simulink model "Microgrid_transition_model_092221"  (R2020a)
settings: Solver=VariableStepAuto  StartTime=0.0  StopTime=16  MaxStep=1e-4  RelTol=1e-3
PreLoadFcn:
  | %run('FC_microgrid_param.m')
  | %load('gen_grid_init.mat')
InitFcn:
  | %load myisoModel_init;
  | run('FC_microgrid_param.m')
  | tic
  | run('CARTinitFcn.m')
  | %caseNo = 2;
  | 
  | %if (caseNo == 1)
  | %set_param(['Isolated_grid_paper_model_022521/SignalGen'], 'ActiveScenario', 'PStep222kW');
  | %else
  | %set_param(['Isolated_grid_paper_model_022521/SignalGen'], 'ActiveScenario', 'QStep222kVAr');
  | 
  | %end;
StopFcn:
  | toc
undefined symbols (not defined in the file): breakpoints1, breakpoints2, cp_table_data, ctrl, D1, Delta, DiscIntNeverNeededParam, DT, FC_BESS, find_system, gcbh, libFC_BESS, LowerLimit, magnitude, oversize, pq_ts, sps_rtmsupport, timer, ts, Ts, Ts_APC, Ts_Control, Ts_Power, UpperLimit
libraries: powerlib x120, powerlib_meascontrol x85, simulink x63, powerlib_extras x40, simulink_extras x12, eePowerMeasurement x9, sps_avr x7, pi_ctrl x4, spsDieselMotorModel x3, SignalEditorBlockLib x2, libLgBattery x1, libFC_PV x1
(part 6 of 11)

== system Microgrid_transition_model_092221/Defferable Load (0-446.25 kW)/Switches/Switches ABC5 ==
  P_ABC : Inport
  Demux : Demux  Outputs=3
      settings: DisplayOption=none
  Switch A : powerlib/Power Electronics/Ideal Switch  Ron=Ron_switch  Lon=0  IC=Status(6)  Rs=Rs_snubber  Cs=Cs_snubber  Measurements=off
      settings: AttributesFormatString=\n  SourceProductBaseCode=MT,PS
  Switch B : powerlib/Power Electronics/Ideal Switch  Ron=Ron_switch  Lon=0  IC=Status(6)  Rs=Rs_snubber  Cs=Cs_snubber  Measurements=off
      settings: AttributesFormatString=\n  SourceProductBaseCode=MT,PS
  Switch C : powerlib/Power Electronics/Ideal Switch  Ron=Ron_switch  Lon=0  IC=Status(6)  Rs=Rs_snubber  Cs=Cs_snubber  Measurements=off
      settings: AttributesFormatString=\n  SourceProductBaseCode=MT,PS
  A : PMIOPort  Side=Left
  B : PMIOPort  Port=2  Side=Left
  C : PMIOPort  Port=3  Side=Left
  "A " : PMIOPort  Port=4  Side=Right
  "B " : PMIOPort  Port=5  Side=Right
  "C " : PMIOPort  Port=6  Side=Right
  wires:
  Demux/1 -> Switch A/1
  Demux/2 -> Switch B/1
  Demux/3 -> Switch C/1
  P_ABC/1 -> Demux/1
  connections:
  C/RConn1 -- Switch C/LConn1
  B/RConn1 -- Switch B/LConn1
  A/RConn1 -- Switch A/LConn1
  Switch A/RConn1 -- "A "/RConn1
  Switch B/RConn1 -- "B "/RConn1
  Switch C/RConn1 -- "C "/RConn1

== system Microgrid_transition_model_092221/Defferable Load (0-446.25 kW)/Switches/Switches ABC6 ==
  P_ABC : Inport
  Demux : Demux  Outputs=3
      settings: DisplayOption=none
  Switch A : powerlib/Power Electronics/Ideal Switch  Ron=Ron_switch  Lon=0  IC=Status(7)  Rs=Rs_snubber  Cs=Cs_snubber  Measurements=off
      settings: AttributesFormatString=\n  SourceProductBaseCode=MT,PS
  Switch B : powerlib/Power Electronics/Ideal Switch  Ron=Ron_switch  Lon=0  IC=Status(7)  Rs=Rs_snubber  Cs=Cs_snubber  Measurements=off
      settings: AttributesFormatString=\n  SourceProductBaseCode=MT,PS
  Switch C : powerlib/Power Electronics/Ideal Switch  Ron=Ron_switch  Lon=0  IC=Status(7)  Rs=Rs_snubber  Cs=Cs_snubber  Measurements=off
      settings: AttributesFormatString=\n  SourceProductBaseCode=MT,PS
  A : PMIOPort  Side=Left
  B : PMIOPort  Port=2  Side=Left
  C : PMIOPort  Port=3  Side=Left
  "A " : PMIOPort  Port=4  Side=Right
  "B " : PMIOPort  Port=5  Side=Right
  "C " : PMIOPort  Port=6  Side=Right
  wires:
  P_ABC/1 -> Demux/1
  Demux/3 -> Switch C/1
  Demux/2 -> Switch B/1
  Demux/1 -> Switch A/1
  connections:
  Switch C/RConn1 -- "C "/RConn1
  Switch B/RConn1 -- "B "/RConn1
  Switch A/RConn1 -- "A "/RConn1
  A/RConn1 -- Switch A/LConn1
  B/RConn1 -- Switch B/LConn1
  C/RConn1 -- Switch C/LConn1

== system Microgrid_transition_model_092221/Defferable Load (0-446.25 kW)/Switches/Switches ABC7 ==
  P_ABC : Inport
  Demux : Demux  Outputs=3
      settings: DisplayOption=none
  Switch A : powerlib/Power Electronics/Ideal Switch  Ron=Ron_switch  Lon=0  IC=Status(8)  Rs=Rs_snubber  Cs=Cs_snubber  Measurements=off
      settings: AttributesFormatString=\n  SourceProductBaseCode=MT,PS
  Switch B : powerlib/Power Electronics/Ideal Switch  Ron=Ron_switch  Lon=0  IC=Status(8)  Rs=Rs_snubber  Cs=Cs_snubber  Measurements=off
      settings: AttributesFormatString=\n  SourceProductBaseCode=MT,PS
  Switch C : powerlib/Power Electronics/Ideal Switch  Ron=Ron_switch  Lon=0  IC=Status(8)  Rs=Rs_snubber  Cs=Cs_snubber  Measurements=off
      settings: AttributesFormatString=\n  SourceProductBaseCode=MT,PS
  A : PMIOPort  Side=Left
  B : PMIOPort  Port=2  Side=Left
  C : PMIOPort  Port=3  Side=Left
  "A " : PMIOPort  Port=4  Side=Right
  "B " : PMIOPort  Port=5  Side=Right
  "C " : PMIOPort  Port=6  Side=Right
  wires:
  Demux/1 -> Switch A/1
  Demux/2 -> Switch B/1
  Demux/3 -> Switch C/1
  P_ABC/1 -> Demux/1
  connections:
  C/RConn1 -- Switch C/LConn1
  B/RConn1 -- Switch B/LConn1
  A/RConn1 -- Switch A/LConn1
  Switch A/RConn1 -- "A "/RConn1
  Switch B/RConn1 -- "B "/RConn1
  Switch C/RConn1 -- "C "/RConn1

== system Microgrid_transition_model_092221/FC_BESS/SMAInverter/85_SMAControl ==
  Uabc : Inport
  Uabc_inv : Inport  Port=2
  Iabc : Inport  Port=3
  CB_status : Inport  Port=4
  Control : Inport  Port=5
  Bus Creator1 : BusCreator  Inputs=2
  Bus Creator5 : BusCreator  Inputs=1
  Bus Selector : BusSelector  OutputSignals=p_ref,q_ref,f_ref,v_ref,GF_mode
  InvControl : Subsystem  mask{Ts=Ts_Control, Unpp=400, Pn=1e6}
      mask prompts: Ts "Control sample time [s]"; Unpp "Nominal AC voltage [Vpp]"; Pn "Nominal Power [W]"
      mask init:
      | Unom = Unpp / sqrt(3);
      | Inom = Pn/3/Unom;
  Rate Transition{,1..2,4..7,9..10} (9 alike) : RateTransition  Integrity=off  OutPortSampleTime=Ts_Control
  Rate Transition3 : RateTransition  OutPortSampleTime=Ts
  Rate Transition8 : RateTransition  OutPortSampleTime=Ts
  Scope : Scope
  Step : Step  Before=1  After=0  SampleTime=Ts
  Step1 : Step  Time=98  SampleTime=Ts
  Sum : Sum  Inputs=|++
  CtrlOut : Outport
  wires:
  Rate Transition4/1 -> InvControl/5(pref)
  Iabc/1 -> Rate Transition1/1
  Rate Transition2/1 -> InvControl/4(cb_stat)
  Rate Transition1/1 -> InvControl/3(Iabc)
  Rate Transition/1 -> InvControl/1(Uabc)
  Rate Transition8/1 -> Bus Creator5/1  "Close"
  Step/1 -> Sum/1
  InvControl/1(Uabc_ref) -> Rate Transition3/1
  Rate Transition3/1 -> Bus Creator1/1  "Uabc"
  Uabc/1 -> Rate Transition/1
  CB_status/1 -> Rate Transition2/1
  Bus Creator5/1 -> Bus Creator1/2  "ToCB"
  Bus Creator1/1 -> CtrlOut/1
  Bus Selector/1 -> Rate Transition4/1  "<p_ref>"
  Bus Selector/2 -> Rate Transition5/1  "<q_ref>"
  Bus Selector/3 -> Rate Transition6/1  "<f_ref>"
  Bus Selector/4 -> Rate Transition7/1  "<v_ref>"
  Bus Selector/5 -> Rate Transition9/1  "<GF_mode>"
  Rate Transition9/1 -> InvControl/9(GF_mode_en)
  Rate Transition7/1 -> InvControl/8(vref)
  Rate Transition5/1 -> InvControl/6(qref)
  Rate Transition6/1 -> InvControl/7(fref)
  Control/1 -> Bus Selector/1
  Uabc_inv/1 -> Rate Transition10/1
  Rate Transition10/1 -> InvControl/2(Uabc_inv)
  Step1/1 -> Sum/2
  Sum/1 -> Scope/1, Rate Transition8/1

== system Microgrid_transition_model_092221/FC_BESS/SMAInverter/BESS Inverter ==
  ctrl : Inport
  Controlled Voltage Source : powerlib/Electrical Sources/Controlled Voltage Source  Initialize=on  Source_Type=AC  Amplitude=0  Phase=0  Frequency=0  Measurements=None
  Controlled Voltage Source1 : powerlib/Electrical Sources/Controlled Voltage Source  Initialize=on  Source_Type=AC  Amplitude=0  Phase=0  Frequency=0  Measurements=None
  Controlled Voltage Source2 : powerlib/Electrical Sources/Controlled Voltage Source  Initialize=on  Source_Type=AC  Amplitude=0  Phase=0  Frequency=0  Measurements=None
  Demux : Demux  Outputs=3
  A : PMIOPort  Side=Right
  N : PMIOPort  Port=2  Side=Left
  B : PMIOPort  Port=3  Side=Right
  C : PMIOPort  Port=4  Side=Right
  wires:
  ctrl/1 -> Demux/1
  Demux/3 -> Controlled Voltage Source2/1
  Demux/2 -> Controlled Voltage Source1/1
  Demux/1 -> Controlled Voltage Source/1
  connections:
  Controlled Voltage Source2/RConn1 -- C/RConn1
  Controlled Voltage Source1/RConn1 -- B/RConn1
  N/RConn1 -- Controlled Voltage Source1/LConn1 -- Controlled Voltage Source/LConn1 -- Controlled Voltage Source2/LConn1
  A/RConn1 -- Controlled Voltage Source/RConn1

== system Microgrid_transition_model_092221/FC_BESS/SMAInverter/Subsystem ==
  GRI1 : powerlib/Measurements/Three-Phase V-I Measurement  VoltageMeasurement=phase-to-ground  SetLabelV=off  LabelV=Ugri  Vpu=off  VpuLL=off  CurrentMeasurement=yes  SetLabelI=off  LabelI=Igri  Ipu=off  Pbase=100e6  Vbase=500e3  OutputType=Complex  PhasorSimulation=off  PSBequivalent=0
  A : PMIOPort  Side=Left
  B : PMIOPort  Port=2  Side=Left
  a : PMIOPort  Port=3  Side=Right
  b : PMIOPort  Port=4  Side=Right
  C : PMIOPort  Port=5  Side=Left
  c : PMIOPort  Port=6  Side=Right
  tag scope: Igri=scoped, Ugri=scoped
  wires:
  GRI1/2 -> [Igri]
  GRI1/1 -> [Ugri]
  connections:
  GRI1/RConn1 -- a/RConn1
  GRI1/LConn1 -- A/RConn1
  GRI1/RConn2 -- b/RConn1
  GRI1/RConn3 -- c/RConn1
  GRI1/LConn2 -- B/RConn1
  GRI1/LConn3 -- C/RConn1

== system Microgrid_transition_model_092221/FC_BESS/SMAInverter/Subsystem1 ==
  SmaINV : powerlib/Measurements/Three-Phase V-I Measurement  VoltageMeasurement=phase-to-ground  SetLabelV=off  LabelV=circuit_Usmainv  Vpu=off  VpuLL=off  CurrentMeasurement=yes  SetLabelI=off  LabelI=circuit_Ismainv  Ipu=off  Pbase=100e6  Vbase=500e3  OutputType=Complex  PhasorSimulation=off  PSBequivalent=0
  A : PMIOPort  Side=Left
  a : PMIOPort  Port=2  Side=Right
  B : PMIOPort  Port=3  Side=Left
  b : PMIOPort  Port=4  Side=Right
  C : PMIOPort  Port=5  Side=Left
  c : PMIOPort  Port=6  Side=Right
  tag scope: Iinv=scoped, Uinv=scoped
  wires:
  SmaINV/1 -> [Uinv]
  SmaINV/2 -> [Iinv]
  connections:
  SmaINV/RConn1 -- a/RConn1
  C/RConn1 -- SmaINV/LConn3
  SmaINV/LConn2 -- B/RConn1
  SmaINV/RConn2 -- b/RConn1
  SmaINV/RConn3 -- c/RConn1
  A/RConn1 -- SmaINV/LConn1

== system Microgrid_transition_model_092221/Grid Feeder Protective Relay/CS Modified PLL/Controller ==
  note: Pierre Giroux, Gilbert Sybille
      | Power System Simulation Laboratory
      | IREQ, Hydro-Quebc
  note: Discrete PID Controller
  Error : Inport
  Discrete Derivative : simulink/Discrete/Discrete Derivative  gainval=1.0  ICPrevScaledInput=0.0  OutMin=[]  OutMax=[]  OutDataType=sfix(16)  OutScaling=2^-10  DoSatur=off
  Discrete-Time Integrator : DiscreteIntegrator  InitialCondition=Init  SampleTime=Ts  LimitOutput=on  UpperSaturationLimit=UpperLimit  LowerSaturationLimit=LowerLimit  ICPrevOutput=DiscIntNeverNeededParam  ICPrevScaledInput=DiscIntNeverNeededParam
  Kp4 : Gain  Gain=Kp  SaturateOnIntegerOverflow=on  OutDataTypeStr=Inherit: Same as input  ParamDataTypeStr=Inherit: Same as input
  Kp5 : Gain  Gain=Ki  SaturateOnIntegerOverflow=on  OutDataTypeStr=Inherit: Same as input  ParamDataTypeStr=Inherit: Same as input
  Kp6 : Gain  Gain=Kd  SaturateOnIntegerOverflow=on  OutDataTypeStr=Inherit: Same as input  ParamDataTypeStr=Inherit: Same as input
  Saturation2 : Saturate  UpperLimit=UpperLimit  LowerLimit=LowerLimit
  Sum6 : Sum  Inputs=+++  InputSameDT=on  SaturateOnIntegerOverflow=on  OutDataTypeStr=Inherit: Same as first input
  Zero-Order Hold : ZeroOrderHold  SampleTime=Ts
  Out : Outport  InitialOutput=0
  wires:
  Error/1 -> Kp4/1, Kp5/1, Kp6/1
  Sum6/1 -> Saturation2/1
  Kp5/1 -> Discrete-Time Integrator/1
  Kp6/1 -> Zero-Order Hold/1
  Kp4/1 -> Sum6/1
  Discrete-Time Integrator/1 -> Sum6/2
  Discrete Derivative/1 -> Sum6/3
  Saturation2/1 -> Out/1
  Zero-Order Hold/1 -> Discrete Derivative/1

== system Microgrid_transition_model_092221/Grid Feeder Protective Relay/CS Modified PLL/VCO ==
  w : Inport
  Compare To Constant : simulink/Logic and Bit Operations/Compare To Constant  relop=>=  const=pi  OutDataTypeStr=uint8
  Gain : Gain  Gain=2*pi  OutDataTypeStr=double
  Gain2 : Gain  Gain=Ts  SaturateOnIntegerOverflow=on  OutDataTypeStr=Inherit: Same as input  ParamDataTypeStr=Inherit: Same as input
  Sum : Sum  Inputs=-++
  Unit Delay1 : UnitDelay  SampleTime=-1  HasFrameUpgradeWarning=on
  theta : Outport
  wires:
  w/1 -> Gain2/1
  Gain/1 -> Sum/1
  Compare To Constant/1 -> Gain/1
  Unit Delay1/1 -> Compare To Constant/1, Sum/3, theta/1  "wt"
  Gain2/1 -> Sum/2
  Sum/1 -> Unit Delay1/1

== system Microgrid_transition_model_092221/Grid Feeder Protective Relay/CS Modified PLL1/Controller ==
  note: Pierre Giroux, Gilbert Sybille
      | Power System Simulation Laboratory
      | IREQ, Hydro-Quebc
  note: Discrete PID Controller
  Error : Inport
  Discrete Derivative : simulink/Discrete/Discrete Derivative  gainval=1.0  ICPrevScaledInput=0.0  OutMin=[]  OutMax=[]  OutDataType=sfix(16)  OutScaling=2^-10  DoSatur=off
  Discrete-Time Integrator : DiscreteIntegrator  InitialCondition=Init  SampleTime=Ts  LimitOutput=on  UpperSaturationLimit=UpperLimit  LowerSaturationLimit=LowerLimit  ICPrevOutput=DiscIntNeverNeededParam  ICPrevScaledInput=DiscIntNeverNeededParam
  Kp4 : Gain  Gain=Kp  SaturateOnIntegerOverflow=on  OutDataTypeStr=Inherit: Same as input  ParamDataTypeStr=Inherit: Same as input
  Kp5 : Gain  Gain=Ki  SaturateOnIntegerOverflow=on  OutDataTypeStr=Inherit: Same as input  ParamDataTypeStr=Inherit: Same as input
  Kp6 : Gain  Gain=Kd  SaturateOnIntegerOverflow=on  OutDataTypeStr=Inherit: Same as input  ParamDataTypeStr=Inherit: Same as input
  Saturation2 : Saturate  UpperLimit=UpperLimit  LowerLimit=LowerLimit
  Sum6 : Sum  Inputs=+++  InputSameDT=on  SaturateOnIntegerOverflow=on  OutDataTypeStr=Inherit: Same as first input
  Zero-Order Hold : ZeroOrderHold  SampleTime=Ts
  Out : Outport  InitialOutput=0
  wires:
  Error/1 -> Kp4/1, Kp5/1, Kp6/1
  Sum6/1 -> Saturation2/1
  Kp5/1 -> Discrete-Time Integrator/1
  Kp6/1 -> Zero-Order Hold/1
  Kp4/1 -> Sum6/1
  Discrete-Time Integrator/1 -> Sum6/2
  Discrete Derivative/1 -> Sum6/3
  Saturation2/1 -> Out/1
  Zero-Order Hold/1 -> Discrete Derivative/1

== system Microgrid_transition_model_092221/Grid Feeder Protective Relay/CS Modified PLL1/VCO ==
  w : Inport
  Compare To Constant : simulink/Logic and Bit Operations/Compare To Constant  relop=>=  const=pi  OutDataTypeStr=uint8
  Gain : Gain  Gain=2*pi  OutDataTypeStr=double
  Gain2 : Gain  Gain=Ts  SaturateOnIntegerOverflow=on  OutDataTypeStr=Inherit: Same as input  ParamDataTypeStr=Inherit: Same as input
  Sum : Sum  Inputs=-++
  Unit Delay1 : UnitDelay  SampleTime=-1  HasFrameUpgradeWarning=on
  theta : Outport
  wires:
  w/1 -> Gain2/1
  Gain/1 -> Sum/1
  Compare To Constant/1 -> Gain/1
  Unit Delay1/1 -> Compare To Constant/1, Sum/3, theta/1  "wt"
  Gain2/1 -> Sum/2
  Sum/1 -> Unit Delay1/1

== system Microgrid_transition_model_092221/Grid Feeder Protective Relay/R25 - Sync Check v0.1/Freq_Comparator ==
  note: This block compares the frequency at the circuit breaker terminals
      | * if the difference is less than threshold dF_threshold, then outputs 1
  f_grid : Inport
  f_gen : Inport  Port=2
  dF_threshold : Inport  Port=3
  Fcn2 : Fcn  Expr=abs(u(2)-u(1)) <= u(3)
  Mux1 : Mux  Inputs=3
  Sum : Sum  Inputs=+-
  Locked : Outport
  dF : Outport  Port=2
  wires:
  Sum/1 -> dF/1
  f_grid/1 -> Mux1/1, Sum/2
  f_gen/1 -> Mux1/2, Sum/1
  dF_threshold/1 -> Mux1/3
  Fcn2/1 -> Locked/1
  Mux1/1 -> Fcn2/1

== system Microgrid_transition_model_092221/Grid Feeder Protective Relay/R25 - Sync Check v0.1/Phase_Comparator ==
  note: This block compares the angle (phase A only) at the circuit breaker terminals
      | * if the difference is less than threshold angle_threshold, then outputs 1
  wt_grid : Inport
  wt_gen : Inport  Port=2
  angle_threshold : Inport  Port=3
  Abs : Abs
  Fcn1 : Fcn  Expr=u(1) <= u(2)  SampleTime=Ts
  Mux1 : Mux  Inputs=2
  Radians to Degrees : simulink_extras/Transformations/Radians to Degrees
  Scope : Scope
  Sum1 : Sum  Inputs=|-+
  WrapPi : Subsystem
  Locked : Outport
  dWt : Outport  Port=2
  wires:
  WrapPi/1(Out1) -> Abs/1, dWt/1
  Sum1/1 -> WrapPi/1(In1)
  wt_grid/1 -> Sum1/1
  wt_gen/1 -> Sum1/2
  Radians to Degrees/1 -> Scope/1, Mux1/1  "R2D"
  Mux1/1 -> Fcn1/1
  angle_threshold/1 -> Mux1/2
  Fcn1/1 -> Locked/1  "bool"
  Abs/1 -> Radians to Degrees/1  "diff"

== system Microgrid_transition_model_092221/Grid Feeder Protective Relay/R25 - Sync Check v0.1/Voltage_Comparator ==
  note: This block compares the voltage at the circuit breaker terminals
      | * if the difference is less than threshold, then outputs 1
  note: dV_threshold% of the nominal VRMSLL
  V_bus : Inport
  V_line : Inport  Port=2
  dV_threshold : Inport  Port=3
  Fcn2 : Fcn  Expr=abs(u(2)-u(1)) <= u(3)
  Mux1 : Mux  Inputs=3
  Sum : Sum  Inputs=+-
  Locked : Outport
  dV : Outport  Port=2
  wires:
  Sum/1 -> dV/1
  dV_threshold/1 -> Mux1/3  "[%]"
  V_bus/1 -> Sum/2, Mux1/1
  V_line/1 -> Mux1/2, Sum/1
  Fcn2/1 -> Locked/1  "thshld"
  Mux1/1 -> Fcn2/1

== system Microgrid_transition_model_092221/Grid Feeder Protective Relay1/CS Modified PLL/Controller ==
  note: Discrete PID Controller
  note: Pierre Giroux, Gilbert Sybille
      | Power System Simulation Laboratory
      | IREQ, Hydro-Quebc
  Error : Inport
  Discrete Derivative : simulink/Discrete/Discrete Derivative  gainval=1.0  ICPrevScaledInput=0.0  OutMin=[]  OutMax=[]  OutDataType=sfix(16)  OutScaling=2^-10  DoSatur=off
  Discrete-Time Integrator : DiscreteIntegrator  InitialCondition=Init  SampleTime=Ts  LimitOutput=on  UpperSaturationLimit=UpperLimit  LowerSaturationLimit=LowerLimit  ICPrevOutput=DiscIntNeverNeededParam  ICPrevScaledInput=DiscIntNeverNeededParam
  Kp4 : Gain  Gain=Kp  SaturateOnIntegerOverflow=on  OutDataTypeStr=Inherit: Same as input  ParamDataTypeStr=Inherit: Same as input
  Kp5 : Gain  Gain=Ki  SaturateOnIntegerOverflow=on  OutDataTypeStr=Inherit: Same as input  ParamDataTypeStr=Inherit: Same as input
  Kp6 : Gain  Gain=Kd  SaturateOnIntegerOverflow=on  OutDataTypeStr=Inherit: Same as input  ParamDataTypeStr=Inherit: Same as input
  Saturation2 : Saturate  UpperLimit=UpperLimit  LowerLimit=LowerLimit
  Sum6 : Sum  Inputs=+++  InputSameDT=on  SaturateOnIntegerOverflow=on  OutDataTypeStr=Inherit: Same as first input
  Zero-Order Hold : ZeroOrderHold  SampleTime=Ts
  Out : Outport  InitialOutput=0
  wires:
  Zero-Order Hold/1 -> Discrete Derivative/1
  Saturation2/1 -> Out/1
  Discrete Derivative/1 -> Sum6/3
  Discrete-Time Integrator/1 -> Sum6/2
  Kp4/1 -> Sum6/1
  Kp6/1 -> Zero-Order Hold/1
  Kp5/1 -> Discrete-Time Integrator/1
  Sum6/1 -> Saturation2/1
  Error/1 -> Kp6/1, Kp5/1, Kp4/1

== system Microgrid_transition_model_092221/Grid Feeder Protective Relay1/CS Modified PLL/VCO ==
  w : Inport
  Compare To Constant : simulink/Logic and Bit Operations/Compare To Constant  relop=>=  const=pi  OutDataTypeStr=uint8
  Gain : Gain  Gain=2*pi  OutDataTypeStr=double
  Gain2 : Gain  Gain=Ts  SaturateOnIntegerOverflow=on  OutDataTypeStr=Inherit: Same as input  ParamDataTypeStr=Inherit: Same as input
  Sum : Sum  Inputs=-++
  Unit Delay1 : UnitDelay  SampleTime=-1  HasFrameUpgradeWarning=on
  theta : Outport
  wires:
  Sum/1 -> Unit Delay1/1
  Gain2/1 -> Sum/2
  Unit Delay1/1 -> theta/1, Sum/3, Compare To Constant/1  "wt"
  Compare To Constant/1 -> Gain/1
  Gain/1 -> Sum/1
  w/1 -> Gain2/1

== system Microgrid_transition_model_092221/Grid Feeder Protective Relay1/CS Modified PLL1/Controller ==
  note: Discrete PID Controller
  note: Pierre Giroux, Gilbert Sybille
      | Power System Simulation Laboratory
      | IREQ, Hydro-Quebc
  Error : Inport
  Discrete Derivative : simulink/Discrete/Discrete Derivative  gainval=1.0  ICPrevScaledInput=0.0  OutMin=[]  OutMax=[]  OutDataType=sfix(16)  OutScaling=2^-10  DoSatur=off
  Discrete-Time Integrator : DiscreteIntegrator  InitialCondition=Init  SampleTime=Ts  LimitOutput=on  UpperSaturationLimit=UpperLimit  LowerSaturationLimit=LowerLimit  ICPrevOutput=DiscIntNeverNeededParam  ICPrevScaledInput=DiscIntNeverNeededParam
  Kp4 : Gain  Gain=Kp  SaturateOnIntegerOverflow=on  OutDataTypeStr=Inherit: Same as input  ParamDataTypeStr=Inherit: Same as input
  Kp5 : Gain  Gain=Ki  SaturateOnIntegerOverflow=on  OutDataTypeStr=Inherit: Same as input  ParamDataTypeStr=Inherit: Same as input
  Kp6 : Gain  Gain=Kd  SaturateOnIntegerOverflow=on  OutDataTypeStr=Inherit: Same as input  ParamDataTypeStr=Inherit: Same as input
  Saturation2 : Saturate  UpperLimit=UpperLimit  LowerLimit=LowerLimit
  Sum6 : Sum  Inputs=+++  InputSameDT=on  SaturateOnIntegerOverflow=on  OutDataTypeStr=Inherit: Same as first input
  Zero-Order Hold : ZeroOrderHold  SampleTime=Ts
  Out : Outport  InitialOutput=0
  wires:
  Zero-Order Hold/1 -> Discrete Derivative/1
  Saturation2/1 -> Out/1
  Discrete Derivative/1 -> Sum6/3
  Discrete-Time Integrator/1 -> Sum6/2
  Kp4/1 -> Sum6/1
  Kp6/1 -> Zero-Order Hold/1
  Kp5/1 -> Discrete-Time Integrator/1
  Sum6/1 -> Saturation2/1
  Error/1 -> Kp6/1, Kp5/1, Kp4/1

== system Microgrid_transition_model_092221/Grid Feeder Protective Relay1/CS Modified PLL1/VCO ==
  w : Inport
  Compare To Constant : simulink/Logic and Bit Operations/Compare To Constant  relop=>=  const=pi  OutDataTypeStr=uint8
  Gain : Gain  Gain=2*pi  OutDataTypeStr=double
  Gain2 : Gain  Gain=Ts  SaturateOnIntegerOverflow=on  OutDataTypeStr=Inherit: Same as input  ParamDataTypeStr=Inherit: Same as input
  Sum : Sum  Inputs=-++
  Unit Delay1 : UnitDelay  SampleTime=-1  HasFrameUpgradeWarning=on
  theta : Outport
  wires:
  Sum/1 -> Unit Delay1/1
  Gain2/1 -> Sum/2
  Unit Delay1/1 -> theta/1, Sum/3, Compare To Constant/1  "wt"
  Compare To Constant/1 -> Gain/1
  Gain/1 -> Sum/1
  w/1 -> Gain2/1

== system Microgrid_transition_model_092221/Grid Feeder Protective Relay1/R25 - Sync Check v0.1/Freq_Comparator ==
  note: This block compares the frequency at the circuit breaker terminals
      | * if the difference is less than threshold dF_threshold, then outputs 1
  f_grid : Inport
  f_gen : Inport  Port=2
  dF_threshold : Inport  Port=3
  Fcn2 : Fcn  Expr=abs(u(2)-u(1)) <= u(3)
  Mux1 : Mux  Inputs=3
  Sum : Sum  Inputs=+-
  Locked : Outport
  dF : Outport  Port=2
  wires:
  Mux1/1 -> Fcn2/1
  Fcn2/1 -> Locked/1
  dF_threshold/1 -> Mux1/3
  f_gen/1 -> Sum/1, Mux1/2
  f_grid/1 -> Sum/2, Mux1/1
  Sum/1 -> dF/1

== system Microgrid_transition_model_092221/Grid Feeder Protective Relay1/R25 - Sync Check v0.1/Phase_Comparator ==
  note: This block compares the angle (phase A only) at the circuit breaker terminals
      | * if the difference is less than threshold angle_threshold, then outputs 1
  wt_grid : Inport
  wt_gen : Inport  Port=2
  angle_threshold : Inport  Port=3
  Abs : Abs
  Fcn1 : Fcn  Expr=u(1) <= u(2)  SampleTime=Ts
  Mux1 : Mux  Inputs=2
  Radians to Degrees : simulink_extras/Transformations/Radians to Degrees
  Scope : Scope
  Sum1 : Sum  Inputs=|-+
  WrapPi : Subsystem
  Locked : Outport
  dWt : Outport  Port=2
  wires:
  Abs/1 -> Radians to Degrees/1  "diff"
  Fcn1/1 -> Locked/1  "bool"
  angle_threshold/1 -> Mux1/2
  Mux1/1 -> Fcn1/1
  Radians to Degrees/1 -> Scope/1, Mux1/1  "R2D"
  wt_gen/1 -> Sum1/2
  wt_grid/1 -> Sum1/1
  Sum1/1 -> WrapPi/1(In1)
  WrapPi/1(Out1) -> dWt/1, Abs/1

== system Microgrid_transition_model_092221/Grid Feeder Protective Relay1/R25 - Sync Check v0.1/Voltage_Comparator ==
  note: dV_threshold% of the nominal VRMSLL
  note: This block compares the voltage at the circuit breaker terminals
      | * if the difference is less than threshold, then outputs 1
  V_bus : Inport
  V_line : Inport  Port=2
  dV_threshold : Inport  Port=3
  Fcn2 : Fcn  Expr=abs(u(2)-u(1)) <= u(3)
  Mux1 : Mux  Inputs=3
  Sum : Sum  Inputs=+-
  Locked : Outport
  dV : Outport  Port=2
  wires:
  Mux1/1 -> Fcn2/1
  Fcn2/1 -> Locked/1  "thshld"
  V_line/1 -> Sum/1, Mux1/2
  V_bus/1 -> Mux1/1, Sum/2
  dV_threshold/1 -> Mux1/3  "[%]"
  Sum/1 -> dV/1

== system Microgrid_transition_model_092221/Wind Turbine Type 4/APC (atomic)1/Baseline ==
  Action Port : ActionPort  ActionPortLabel=case [ 5 ]:
  Constant1 : Constant  Value=0
  Qcmd : Outport
  dP : Outport  Port=2
  dT : Outport  Port=3
  wires:
  Constant1/1 -> dP/1, dT/1, Qcmd/1

== system Microgrid_transition_model_092221/Wind Turbine Type 4/APC (atomic)1/Inertial Response (to df) ==
  Freq (Hz) : Inport
  type1 : Inport  Port=2
  wg (pu) : Inport  Port=3
  Action Port : ActionPort  ActionPortLabel=case [ 1 ]:
  Constant1 : Constant  Value=0
  Constant2 : Constant  Value=0
  Constant3 : Constant  Value=1e-3
  Constant4 : Constant  Value=60
  Display{3..4,6..7} (4 alike) : Display
  Divide1 : Product  Inputs=*/
  FBIC : Subsystem
  Lock2 : Subsystem
  Rate Limiter1 : RateLimiter  RisingSlewLimit=0.45  SampleTimeMode=inherited
  Relational Operator3 : RelationalOperator  OutDataTypeStr=boolean  RndMeth=Nearest
  Relational Operator4 : RelationalOperator  Operator=<=  OutDataTypeStr=boolean  RndMeth=Nearest
  Saturation : Saturate  UpperLimit=0.4  LowerLimit=0
  Saturation1 : Saturate  UpperLimit=1  LowerLimit=1e-5
  Scope : Scope  NumInputPorts=3
  Sum1 : Sum  Inputs=|-+
  Switch1 : Switch  Criteria=u2 > Threshold  Threshold=1
  TLIC : Subsystem  TreatAsAtomicUnit=on
  Type1 : Switch  Criteria=u2 > Threshold  Threshold=0.5
  When to start IR : DigitalClock  SampleTime=-1
  dead band1 : Constant  Value=0.2
  dT : Outport
  dP : Outport  Port=2
  Qcmd : Outport  Port=3
  wires:
  Constant1/1 -> dP/1, Qcmd/1
  Constant2/1 -> Switch1/3
  When to start IR/1 -> Switch1/2
  Lock2/1(O) -> Switch1/1
  Saturation/1 -> dT/1
  wg (pu)/1 -> [Wg], FBIC/1(wg (pu))
  Switch1/1 -> Display3/1, Scope/3, [In_Act]
  type1/1 -> Type1/2
  Sum1/1 -> Relational Operator3/1, Scope/2
  FBIC/1(Delta_P FBIC1) -> Type1/3
  Type1/1 -> [Delta_P], Display6/1
  Freq (Hz)/1 -> FBIC/2(Freq (Hz)1), [Freq]
  [In_Act] -> FBIC/3(Act1), TLIC/1(Act)
  TLIC/1(Delta_P TLIC) -> Type1/1
  [Delta_P] -> Relational Operator4/1
  Constant4/1 -> Sum1/2
  dead band1/1 -> Relational Operator3/2
  Divide1/1 -> Rate Limiter1/1
  [Wg] -> Saturation1/1
  Saturation1/1 -> Divide1/2
  Constant3/1 -> Relational Operator4/2
  Relational Operator4/1 -> Display7/1, Lock2/2(R)
  [Freq] -> Sum1/1, Display4/1
  [Delta_P] -> Divide1/1, Scope/1
  Relational Operator3/1 -> Lock2/1(I)
  Rate Limiter1/1 -> Saturation/1

== system Microgrid_transition_model_092221/Wind Turbine Type 4/APC (atomic)1/PFR ==
  Freq (Hz) : Inport
  Action Port : ActionPort  ActionPortLabel=case [ 2 ]:
  Constant1 : Constant  Value=0
  Constant2 : Constant  Commented=on  Value=-1
  Constant3 : Constant  Value=60
  Dead Zone : DeadZone  LowerValue=-db/60  UpperValue=db/60  SaturateOnIntegerOverflow=on
  Divide1 : Product  Inputs=*/
  P/f gain : Gain  Gain=1/k
  Saturation : Saturate  UpperLimit=0
  Sum : Sum  Inputs=|+-
  Sum1 : Sum  Inputs=|-+
  Switch1 : Switch  Commented=on  Criteria=u2 > Threshold  Threshold=57
  curtailment pu : Constant  Value=0.2
  dP : Outport
  dT : Outport  Port=2
  Qcmd : Outport  Port=3
  wires:
  ? -> Switch1/2
  Constant2/1 -> Switch1/3
  Sum/1 -> Saturation/1
  Constant1/1 -> dT/1, Qcmd/1
  Saturation/1 -> dP/1
  P/f gain/1 -> Sum/1
  curtailment pu/1 -> Sum/2
  Dead Zone/1 -> P/f gain/1
  Constant3/1 -> Sum1/2, Divide1/2
  Freq (Hz)/1 -> Sum1/1
  Divide1/1 -> Dead Zone/1  "delta f pu"
  Sum1/1 -> Divide1/1

== system Microgrid_transition_model_092221/Wind Turbine Type 4/APC (atomic)1/PQ ==
  SFRcmd : Inport
  Qin : Inport  Port=2
  Action Port : ActionPort  ActionPortLabel=case [ 3 ]:
  Constant : Constant
  Constant1 : Constant  Value=0
  Sum : Sum  Inputs=|+-
  dP : Outport
  Qcmd : Outport  Port=2
  dT : Outport  Port=3
  wires:
  Constant1/1 -> dT/1
  Qin/1 -> Qcmd/1
  Constant/1 -> Sum/2
  Sum/1 -> dP/1
  SFRcmd/1 -> Sum/1

== system Microgrid_transition_model_092221/Wind Turbine Type 4/APC (atomic)1/VR (handled by FRT) ==
  Action Port : ActionPort  ActionPortLabel=case [ 4 ]:
  Constant1 : Constant  Value=0
  Qcmd : Outport
  dP : Outport  Port=2
  dT : Outport  Port=3
  wires:
  Constant1/1 -> Qcmd/1, dT/1, dP/1

== system Microgrid_transition_model_092221/Wind Turbine Type 4/Control/Excitation Control system ==
  Flux : Inport
  wr : Inport  Port=2
  Discrete PI Controller : Subsystem  DialogController=POWERSYS.PowerSysDialog  mask(Discrete PI Controller){Kp=Kp_field, Ki=Ki_field, Par_Limits=[1 0]*Vf_limit, Init=init(9), Ts=Ts}
      mask prompts: Kp "Proportional gain (Kp):"; Ki "Integral gain (Ki):"; Par_Limits "Output limits: [ Upper   Lower ]"; Init "Output initial value:"; Ts "Sample time:"
      mask help: This block implements a discrete PI controller.
      mask init:
      | UpperLimit=Par_Limits(1);
      | LowerLimit=Par_Limits(2);
      | power_initmask();
      mask Help: This block is part of a subset of blocks in the Extras library that does not have documentation associated with it, other than the block mask description.
      mask Display: disp('PI');
  Divide : Product  Inputs=*/
  Flux_ref : Constant
  "Flux_ref " : Constant
  Sum4 : Sum  Inputs=|+-  InputSameDT=on  SaturateOnIntegerOverflow=on  OutDataTypeStr=Inherit: Same as first input
  Switch : Switch  Threshold=1
  avoid division by 0 : Saturate  UpperLimit=inf  LowerLimit=1e-6
  Vf : Outport  VectorParamsAs1DForOutWhenUnconnected=off
  wires:
  Sum4/1 -> Discrete PI Controller/1(Error)
  Discrete PI Controller/1(Out) -> Vf/1  "Vf"
  Flux/1 -> Sum4/2  "Flux"
  wr/1 -> Switch/2, avoid division by 0/1
  Flux_ref/1 -> Switch/3
  "Flux_ref "/1 -> Divide/1
  avoid division by 0/1 -> Divide/2
  Divide/1 -> Switch/1
  Switch/1 -> Sum4/1
